simulink model "sampleModel68"  (R2021b)
settings: Solver=VariableStepAuto  StartTime=0.0  StopTime=10.0  RelTol=1e-3
undefined symbols (not defined in the file or in its folder): magnitude, Newton, Raphson
libraries: simulink x9, slpidlib x2
settings Model: Creator=user  LastModifiedBy=user

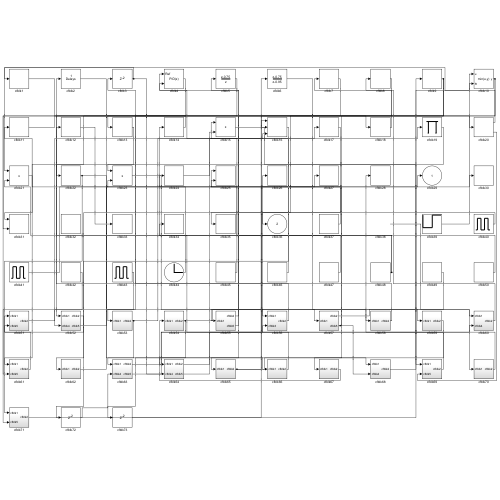
[thumbnail: Simulink's stored preview of the top-level diagram]
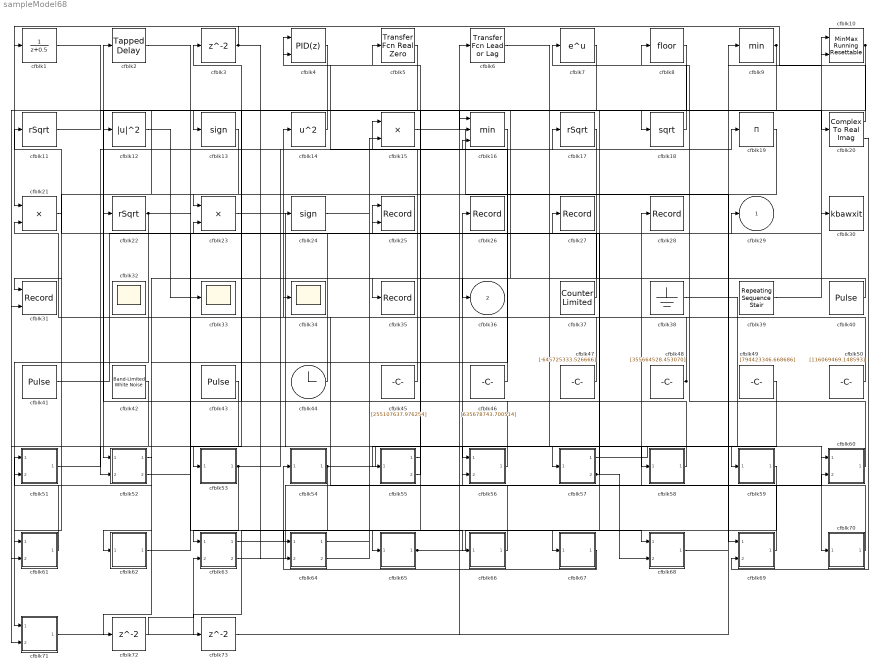
== system sampleModel68 ==
  cfblk1 : DiscreteTransferFcn  SampleTime=1
  cfblk10 : simulink/Math Operations/MinMax Running Resettable  Function=min  vinit=0.0
  cfblk11 : Sqrt  Operator=rSqrt  AlgorithmType=Newton-Raphson  SaturateOnIntegerOverflow=on
  cfblk12 : Math  Operator=magnitude^2  SaturateOnIntegerOverflow=on
  cfblk13 : Signum
  cfblk14 : Math  Operator=square  SaturateOnIntegerOverflow=on
  cfblk15 : Product  Inputs=**
  cfblk16 : MinMax  Inputs=3
  cfblk17 : Sqrt  Operator=rSqrt  AlgorithmType=Newton-Raphson  SaturateOnIntegerOverflow=on
  cfblk18 : Sqrt  SaturateOnIntegerOverflow=on
  cfblk19 : Product  Inputs=*
  cfblk2 : simulink/Discrete/Tapped Delay  vinit=0.0  samptime=-1  NumDelays=1  DelayOrder=Oldest  includeCurrent=off
  cfblk20 : ComplexToRealImag
  cfblk21 : Product
  cfblk22 : Sqrt  Operator=rSqrt  AlgorithmType=Newton-Raphson  SaturateOnIntegerOverflow=on
  cfblk23 : Product  Inputs=**
  cfblk24 : Signum
  cfblk25 : Record  FileSettingsInternal="{\"entries\":[{\"content\":{\"excelSettings\":{\"content\":{},\"type\":\"Streamout.ExcelSettings\"}},\"type\":\"Streamout.FileSettingStorage\",\"uuid\":\"7380ae25-d94a-4681-bf5d-5ee3cf68c672\"}],\"packageUris\":[\"http://schema.mathworks.com/mf0/streamout_blocks/R2020a\"],\"version\":\"1.0\"}"  Layout=[1 1]  SignalsInternal="{\"entries\":[{\"content\":{\"signals\":[{\"content\":{\"blockPath\":[\"sampleModel68/cfblk25\"],\"channel\":[],\"dimensions\":[1],\"domain\":\"sampleModel68/cfblk25\",\"lineColor\":\"#a2142f\",\"plots\":[1],\"port\":1,\"sid\":[\"\"],\"signalID\":2597,\"signalName\":\"cfblk45\"},\"type\":\"RecordBlkView.Signal\",\"uuid\":\"14372fe8-37bd-4dd9-b022-ca2b2938b13a\"},{\"content\":{\"blockPath\":[\"sampleModel68/cfblk25\"],\"channel\":[],\"dimensions\":[1],\"domain\":\"sampleModel68/cfblk25\",\"lineColor\":\"#139fff\",\"plots\":[1],\"port\":2,\"sid\":[\"\"],\"signalID\":2601,\"signalName\":\"cfblk57:2\"},\"type\":\"RecordBlkView.Signal\",\"uuid\":\"d926118c-bf66-4285-a082-df532e1a02d1\"}]},\"type\":\"RecordBlkView.InputSignals\",\"uuid\":\"7acbd860-2b2a-4c58-bd97-e2d0956e5af0\"}],\"packageUris\":[\"http://schema.mathworks.com/mf0/streamout_blocks/R2020a\"],\"version\":\"1.0\"}"  VisualizationBindings="{\"xyplotplugin\":{\"info\":[{\"series\":[{\"bindingParametersList\":[{\"parameter\":\"X-Axis\",\"signalID\":2597,\"signalName\":\"cfblk45\"},{\"parameter\":\"Y-Axis\",\"signalID\":2601,\"signalName\":\"cfblk57:2\"}],\"seriesID\":43011}],\"subplotID\":1}]}}"  CompatibilityTag=XY
  cfblk26 : Record  FileSettingsInternal="{\"entries\":[{\"content\":{\"excelSettings\":{\"content\":{},\"type\":\"Streamout.ExcelSettings\"}},\"type\":\"Streamout.FileSettingStorage\",\"uuid\":\"f47baa91-5e85-4539-9bdd-62570cf60bad\"}],\"packageUris\":[\"http://schema.mathworks.com/mf0/streamout_blocks/R2020a\"],\"version\":\"1.0\"}"  SignalsInternal="{\"entries\":[{\"content\":{\"signals\":[{\"content\":{\"blockPath\":[\"sampleModel68/cfblk26\"],\"channel\":[],\"dimensions\":[1],\"domain\":\"sampleModel68/cfblk26\",\"lineColor\":\"#0072bd\",\"plots\":[1],\"port\":1,\"sid\":[\"\"],\"signalID\":2617,\"signalName\":\"cfblk66\"},\"type\":\"RecordBlkView.Signal\",\"uuid\":\"ce7d10c1-a342-4b76-a021-8b8f96db9006\"}]},\"type\":\"RecordBlkView.InputSignals\",\"uuid\":\"a1fcf589-8043-40eb-83d7-4e4254cbec00\"}],\"packageUris\":[\"http://schema.mathworks.com/mf0/streamout_blocks/R2020a\"],\"version\":\"1.0\"}"  VisualizationBindings="{\"sparklinesplugin\":{\"info\":[{\"bindingParametersList\":[],\"subplotID\":1}]}}"
  cfblk27 : Record  FileSettingsInternal="{\"entries\":[{\"content\":{\"excelSettings\":{\"content\":{},\"type\":\"Streamout.ExcelSettings\"}},\"type\":\"Streamout.FileSettingStorage\",\"uuid\":\"7fca77e6-a95a-4af2-994f-8cefc4879576\"}],\"packageUris\":[\"http://schema.mathworks.com/mf0/streamout_blocks/R2020a\"],\"version\":\"1.0\"}"  SignalsInternal="{\"entries\":[{\"content\":{\"signals\":[{\"content\":{\"blockPath\":[\"sampleModel68/cfblk27\"],\"channel\":[],\"dimensions\":[1],\"domain\":\"sampleModel68/cfblk27\",\"lineColor\":\"#ff13a6\",\"plots\":[1],\"port\":1,\"sid\":[\"\"],\"signalID\":2605,\"signalName\":\"cfblk62\"},\"type\":\"RecordBlkView.Signal\",\"uuid\":\"25dd8e9c-f56c-4ed2-a9cf-a14533026692\"}]},\"type\":\"RecordBlkView.InputSignals\",\"uuid\":\"8aec1518-f338-4448-a462-eff875f2086d\"}],\"packageUris\":[\"http://schema.mathworks.com/mf0/streamout_blocks/R2020a\"],\"version\":\"1.0\"}"  VisualizationBindings="{\"sparklinesplugin\":{\"info\":[{\"bindingParametersList\":[],\"subplotID\":1}]}}"
  cfblk28 : Record  FileSettingsInternal="{\"entries\":[{\"content\":{\"excelSettings\":{\"content\":{},\"type\":\"Streamout.ExcelSettings\"}},\"type\":\"Streamout.FileSettingStorage\",\"uuid\":\"0b6a57c5-e48f-4051-9630-9944b72aff24\"}],\"packageUris\":[\"http://schema.mathworks.com/mf0/streamout_blocks/R2020a\"],\"version\":\"1.0\"}"  SignalsInternal="{\"entries\":[{\"content\":{\"signals\":[{\"content\":{\"blockPath\":[\"sampleModel68/cfblk28\"],\"channel\":[],\"dimensions\":[1],\"domain\":\"sampleModel68/cfblk28\",\"lineColor\":\"#edb120\",\"plots\":[1],\"port\":1,\"sid\":[\"\"],\"signalID\":2625,\"signalName\":\"cfblk70\"},\"type\":\"RecordBlkView.Signal\",\"uuid\":\"dc8e6425-624f-40ca-b929-8e8e8d4940ce\"}]},\"type\":\"RecordBlkView.InputSignals\",\"uuid\":\"d190679b-f694-456f-800b-168cbe042715\"}],\"packageUris\":[\"http://schema.mathworks.com/mf0/streamout_blocks/R2020a\"],\"version\":\"1.0\"}"  VisualizationBindings="{\"sparklinesplugin\":{\"info\":[{\"bindingParametersList\":[],\"subplotID\":1}]}}"
  cfblk3 : Delay  SampleTime=1
  cfblk30 : ToWorkspace  VariableName=kbawxit  SaveFormat=Timeseries  SampleTime=-1
  cfblk31 : Record  FileSettingsInternal="{\"entries\":[{\"content\":{\"excelSettings\":{\"content\":{},\"type\":\"Streamout.ExcelSettings\"}},\"type\":\"Streamout.FileSettingStorage\",\"uuid\":\"7dd7fc0f-01a8-4e3d-a00e-f98f5cc25ed7\"}],\"packageUris\":[\"http://schema.mathworks.com/mf0/streamout_blocks/R2020a\"],\"version\":\"1.0\"}"  Layout=[1 1]  SignalsInternal="{\"entries\":[{\"content\":{\"signals\":[{\"content\":{\"blockPath\":[\"sampleModel68/cfblk31\"],\"channel\":[],\"dimensions\":[1],\"domain\":\"sampleModel68/cfblk31\",\"lineColor\":\"#a2142f\",\"plots\":[1],\"port\":1,\"sid\":[\"\"],\"signalID\":2609,\"signalName\":\"cfblk13\"},\"type\":\"RecordBlkView.Signal\",\"uuid\":\"1befd8ad-63b6-41b6-b49e-12842e72401a\"},{\"content\":{\"blockPath\":[\"sampleModel68/cfblk31\"],\"channel\":[],\"dimensions\":[1],\"domain\":\"sampleModel68/cfblk31\",\"lineColor\":\"#139fff\",\"plots\":[1],\"port\":2,\"sid\":[\"\"],\"signalID\":2613,\"signalName\":\"cfblk4\"},\"type\":\"RecordBlkView.Signal\",\"uuid\":\"e4cc32b6-11bf-4c93-9d61-67df3e9ed535\"}]},\"type\":\"RecordBlkView.InputSignals\",\"uuid\":\"9e53f5fc-b0f2-4e3d-bb43-917b54e9e2d2\"}],\"packageUris\":[\"http://schema.mathworks.com/mf0/streamout_blocks/R2020a\"],\"version\":\"1.0\"}"  VisualizationBindings="{\"xyplotplugin\":{\"info\":[{\"series\":[{\"bindingParametersList\":[{\"parameter\":\"X-Axis\",\"signalID\":2609,\"signalName\":\"cfblk13\"},{\"parameter\":\"Y-Axis\",\"signalID\":2613,\"signalName\":\"cfblk4\"}],\"seriesID\":44428}],\"subplotID\":1}]}}"  CompatibilityTag=XY
  cfblk32 : Scope
      settings: Floating=on
  cfblk33 : Scope
  cfblk34 : Scope
  cfblk35 : Record  FileSettingsInternal="{\"entries\":[{\"content\":{\"excelSettings\":{\"content\":{},\"type\":\"Streamout.ExcelSettings\"}},\"type\":\"Streamout.FileSettingStorage\",\"uuid\":\"e62acdcb-7c93-4ae9-a251-67a68609c7cf\"}],\"packageUris\":[\"http://schema.mathworks.com/mf0/streamout_blocks/R2020a\"],\"version\":\"1.0\"}"  SignalsInternal="{\"entries\":[{\"content\":{\"signals\":[{\"content\":{\"blockPath\":[\"sampleModel68/cfblk35\"],\"channel\":[],\"dimensions\":[1],\"domain\":\"sampleModel68/cfblk35\",\"lineColor\":\"#d95319\",\"plots\":[1],\"port\":1,\"sid\":[\"\"],\"signalID\":2621,\"signalName\":\"cfblk40\"},\"type\":\"RecordBlkView.Signal\",\"uuid\":\"cba5933c-5ebb-4ff9-ad8b-2eadd83d23f5\"}]},\"type\":\"RecordBlkView.InputSignals\",\"uuid\":\"4eef4586-6a89-45b6-bd2f-dfe3524fb43a\"}],\"packageUris\":[\"http://schema.mathworks.com/mf0/streamout_blocks/R2020a\"],\"version\":\"1.0\"}"  VisualizationBindings="{\"sparklinesplugin\":{\"info\":[{\"bindingParametersList\":[],\"subplotID\":1}]}}"
  cfblk37 : simulink/Sources/Counter Limited  uplimit=[649.000000]  tsamp=-1
  cfblk38 : Ground
  cfblk39 : simulink/Sources/Repeating Sequence Stair  OutValues=[645973491.139830, 703038970.892550]  tsamp=-1  OutMin=[]  OutMax=[]  OutDataTypeStr=double  OutputDataTypeScalingMode=double  OutDataType=fixdt(0,8)  ConRadixGroup=Best Precision: Vector-wise  OutScaling=2^-12
  cfblk4 : slpidlib/PID Controller (2DOF)  Controller=PID  Form=Parallel  TimeDomain=Discrete-time  UseExternalTs=off  SampleTime=1  IntegratorMethod=Forward Euler  FilterMethod=Forward Euler  ControllerParametersSource=internal  P=1  I=1  D=0  UseFilter=on  N=100  b=1  c=1  TunerSelectOption=Transfer Function Based (PID Tuner App)  InitialConditionSource=internal  InitialConditionForIntegrator=0  InitialConditionForFilter=0  DifferentiatorICPrevScaledInput=0  ExternalReset=none  TrackingMode=off  Kt=1  LimitOutput=off  SatLimitsSource=internal  UpperSaturationLimit=inf  LowerSaturationLimit=-inf  LinearizeAsGain=off  AntiWindupMode=none  Kb=1  POutMin=[]  POutMax=[]  IOutMin=[]  IOutMax=[]  DOutMin=[]  DOutMax=[]  NOutMin=[]  NOutMax=[]  bOutMin=[]  bOutMax=[]  cOutMin=[]  cOutMax=[]  SumOutMin=[]  SumOutMax=[]  SaturationOutMin=[]  SaturationOutMax=[]  PParamMin=[]  PParamMax=[]  IParamMin=[]  IParamMax=[]  DParamMin=[]  DParamMax=[]  NParamMin=[]  NParamMax=[]  bParamMin=[]  bParamMax=[]  cParamMin=[]  cParamMax=[]  KbParamMin=[]  KbParamMax=[]  KtParamMin=[]  KtParamMax=[]  KbOutMin=[]  KbOutMax=[]  KtOutMin=[]  KtOutMax=[]  IntegratorOutMin=[]  IntegratorOutMax=[]  FilterOutMin=[]  FilterOutMax=[]  SumI1OutMin=[]  SumI1OutMax=[]  SumI2OutMin=[]  SumI2OutMax=[]  SumI3OutMin=[]  SumI3OutMax=[]  SumI4OutMin=[]  SumI4OutMax=[]  SumDOutMin=[]  SumDOutMax=[]  Sum1OutMin=[]  Sum1OutMax=[]  Sum2OutMin=[]  Sum2OutMax=[]  Sum3OutMin=[]  Sum3OutMax=[]  DifferentiatorOutMin=[]  DifferentiatorOutMax=[]  FilterDiffOutCoefMin=[]  FilterDiffOutCoefMax=[]  ReciprocalOutMin=[]  ReciprocalOutMax=[]  SumDenOutMin=[]  SumDenOutMax=[]  SumNumOutMin=[]  SumNumOutMax=[]  DivideOutMin=[]  DivideOutMax=[]  UdiffTsProdOutMin=[]  UdiffTsProdOutMax=[]  NTsProdOutMin=[]  NTsProdOutMax=[]  UintegralTsProdOutMin=[]  UintegralTsProdOutMax=[]  UngainTsProdOutMin=[]  UngainTsProdOutMax=[]  IntegratorContinuousStateAttributes=''  IntegratorStateMustResolveToSignalObject=off  IntegratorRTWStateStorageClass=Auto  FilterContinuousStateAttributes=''  FilterStateMustResolveToSignalObject=off  FilterRTWStateStorageClass=Auto  ParallelPVariant=InternalParameters  IdealPVariant=Disabled  IVariant=InternalParameters  DVariant=InternalParameters  bVariant=InternalParameters  cVariant=InternalParameters  IntegratorVariant=Discrete  SatVariant=Disabled  AWVariant=Passthrough  PCopyVariant=Disabled  TRVariant=Disabled  FdbkBlocksVariant=Forward  IdealPFdbkVariant=Disabled  SatFdbkVariant=Disabled  DerivativeFilterVariant=ForwardEulerFilter  NVariant=InternalParameters  NCopyVariant=Disabled  FilterICVariant=InternalICsFilter  IntegratorICVariant=InternalICs  ExternalResetVariant=Disabled  TRSumVariant=Passthrough  SumFdbkVariant=Disabled  SumVariant=Sum_PID  TsampFilterVariant=InternalTs  TsampNgainVariant=Passthrough  TsampIntegralVariant=Passthrough  ExternalSaturationOutDataTypeStr=Inherit: Same as second input
      settings: SourceProductBaseCode=SL
  cfblk40 : DiscretePulseGenerator  PulseType=Time based  Amplitude=[-445442640.127411]  Period=[11449827.973829]  PulseWidth=5  PhaseDelay=[6.000000]
  cfblk41 : DiscretePulseGenerator  PulseType=Time based  Amplitude=[-687630750.798750]  Period=[5327849.825297]  PulseWidth=5  PhaseDelay=[4.000000]
  cfblk42 : simulink/Sources/Band-Limited White Noise  Cov=[9357779221.486231]  Ts=0.1  seed=[2033079699.000000]
  cfblk43 : DiscretePulseGenerator  PulseType=Time based  Amplitude=[-140736143.976516]  Period=[50342523.627179]  PulseWidth=5  PhaseDelay=[2.000000]
  cfblk44 : Clock
  cfblk45 : Constant  Value=[255107637.976254]  SampleTime=1
  cfblk46 : Constant  Value=[635678743.700514]  SampleTime=1
  cfblk47 : Constant  Value=[-645725333.526666]  SampleTime=1
  cfblk48 : Constant  Value=[355664528.453070]  SampleTime=1
  cfblk49 : Constant  Value=[794423346.668686]  SampleTime=1
  cfblk5 : simulink/Discrete/Transfer Fcn Real Zero  ZeroZ=0.75  ICPrevInput=0.0  DoSatur=off
      settings: SourceProductBaseCode=SL
  cfblk50 : Constant  Value=[116069469.148593]  SampleTime=1
  cfblk51 : Subsystem
  cfblk52 : Subsystem
  cfblk53 : Subsystem
  cfblk54 : Subsystem
  cfblk55 : Subsystem
  cfblk56 : Subsystem
  cfblk57 : Subsystem
  cfblk58 : Subsystem
  cfblk59 : Subsystem
  cfblk6 : simulink/Discrete/Transfer Fcn Lead or Lag  PoleZ=0.95  ZeroZ=0.75  ICPrevOutput=0.0  ICPrevInput=0.0  DoSatur=off
      settings: SourceProductBaseCode=SL
  cfblk60 : Subsystem
  cfblk61 : Subsystem
  cfblk62 : Subsystem
  cfblk63 : Subsystem
  cfblk64 : Subsystem
  cfblk65 : Subsystem
  cfblk66 : Subsystem
  cfblk67 : Subsystem
  cfblk68 : Subsystem
  cfblk69 : Subsystem
  cfblk7 : Math  SaturateOnIntegerOverflow=on
  cfblk70 : Subsystem
  cfblk71 : Subsystem
  cfblk72 : Delay  SampleTime=1
  cfblk73 : Delay  SampleTime=1
  cfblk8 : Rounding
  cfblk9 : MinMax
  cfblk29 : Outport
  cfblk36 : Outport  Port=2
  wires:
  cfblk40/1 -> cfblk35/1
  cfblk66/1(cfblk2) -> cfblk26/1
  cfblk67/1(cfblk2) -> cfblk54/1(cfblk1)
  cfblk12/1 -> cfblk33/1
  cfblk48/1 -> cfblk15/1, cfblk21/2
  cfblk20/1 -> cfblk21/1
  cfblk56/1(cfblk2) -> cfblk2/1
  cfblk50/1 -> cfblk14/1
  cfblk54/1(cfblk2) -> cfblk59/1(cfblk1), cfblk64/1(cfblk1)
  cfblk53/1(cfblk2) -> cfblk63/1(cfblk1), cfblk16/3
  cfblk5/1 -> cfblk52/1(cfblk1)
  cfblk22/1 -> cfblk71/1(cfblk1), cfblk57/1(cfblk1)
  cfblk55/1(cfblk2) -> cfblk5/1
  cfblk42/1 -> cfblk71/2(cfblk5)
  cfblk9/1 -> cfblk36/1, cfblk22/1, cfblk61/2(cfblk5)
  cfblk43/1 -> cfblk52/2(cfblk4)
  cfblk51/1(cfblk2) -> cfblk17/1
  cfblk38/1 -> cfblk70/1(cfblk1)
  cfblk47/1 -> cfblk12/1
  cfblk23/1 -> cfblk56/1(cfblk1)
  cfblk71/1(cfblk2) -> cfblk6/1
  cfblk58/1(cfblk2) -> cfblk3/1
  cfblk69/1(cfblk2) -> cfblk34/1
  cfblk37/1 -> cfblk24/1
  cfblk17/1 -> cfblk62/1(cfblk1)
  cfblk44/1 -> cfblk11/1
  cfblk61/1(cfblk2) -> cfblk51/1(cfblk1)
  cfblk15/1 -> cfblk69/1(cfblk1)
  cfblk3/1 -> cfblk1/1, cfblk64/2(cfblk4)
  cfblk70/1(cfblk2) -> cfblk28/1
  cfblk18/1 -> cfblk7/1
  cfblk63/1(cfblk2) -> cfblk16/1
  cfblk63/2(cfblk5) -> cfblk56/2(cfblk3)
  cfblk21/1 -> cfblk61/1(cfblk1)
  cfblk39/1 -> cfblk10/1
  cfblk45/1 -> cfblk25/1
  cfblk65/1(cfblk2) -> cfblk68/1(cfblk1), cfblk29/1
  cfblk20/2 -> cfblk69/2(cfblk5)
  cfblk6/1 -> cfblk58/1(cfblk1)
  cfblk8/1 -> cfblk16/2
  cfblk2/1 -> cfblk66/1(cfblk1)
  cfblk10/1 -> cfblk55/1(cfblk1), cfblk67/1(cfblk1)
  cfblk57/1(cfblk2) -> cfblk60/1(cfblk1)
  cfblk11/1 -> cfblk20/1
  cfblk64/1(cfblk2) -> cfblk15/2
  cfblk7/1 -> cfblk53/1(cfblk1)
  cfblk13/1 -> cfblk31/1
  cfblk60/1(cfblk2) -> cfblk8/1
  cfblk1/1 -> cfblk18/1
  cfblk46/1 -> cfblk4/1
  cfblk4/1 -> cfblk31/2
  cfblk55/2(cfblk5) -> cfblk4/2
  cfblk19/1 -> cfblk23/1
  cfblk52/1(cfblk2) -> cfblk51/2(cfblk5)
  cfblk49/1 -> cfblk65/1(cfblk1)
  cfblk68/1(cfblk2) -> cfblk10/2
  cfblk14/1 -> cfblk13/1
  cfblk62/1(cfblk2) -> cfblk27/1
  cfblk57/2(cfblk5) -> cfblk25/2, cfblk68/2(cfblk4)
  cfblk41/1 -> cfblk23/2
  cfblk64/2(cfblk5) -> cfblk60/2(cfblk4)
  cfblk24/1 -> cfblk19/1
  cfblk52/2(cfblk5) -> cfblk30/1
  cfblk16/1 -> cfblk72/1
  cfblk72/1 -> cfblk63/2(cfblk4)
  cfblk59/1(cfblk2) -> cfblk73/1
  cfblk73/1 -> cfblk9/1

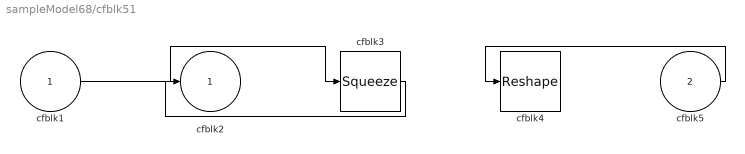
== system sampleModel68/cfblk51 ==
  cfblk1 : Inport
  cfblk5 : Inport  Port=2
  cfblk3 : Squeeze
  cfblk4 : Reshape
  cfblk2 : Outport
  wires:
  cfblk1/1 -> cfblk3/1
  cfblk5/1 -> cfblk4/1
  cfblk3/1 -> cfblk2/1

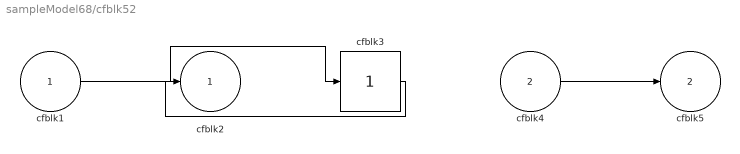
== system sampleModel68/cfblk52 ==
  cfblk1 : Inport
  cfblk4 : Inport  Port=2
  cfblk3 : simulink/Math Operations/Slider Gain  gain=1  low=0  high=2
  cfblk2 : Outport
  cfblk5 : Outport  Port=2
  wires:
  cfblk4/1 -> cfblk5/1
  cfblk1/1 -> cfblk3/1
  cfblk3/1 -> cfblk2/1

== system sampleModel68/cfblk53 ==
  cfblk1 : Inport
  cfblk3 : Delay  SampleTime=1
  cfblk2 : Outport
  wires:
  cfblk1/1 -> cfblk3/1
  cfblk3/1 -> cfblk2/1

== system sampleModel68/cfblk54 ==
  cfblk1 : Inport
  cfblk3 : DiscreteTransferFcn  SampleTime=1
  cfblk2 : Outport
  wires:
  cfblk3/1 -> cfblk2/1
  cfblk1/1 -> cfblk3/1

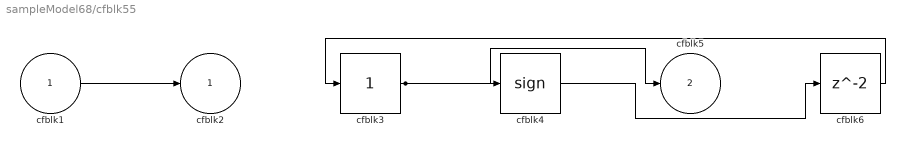
== system sampleModel68/cfblk55 ==
  cfblk1 : Inport
  cfblk3 : simulink/Math Operations/Slider Gain  gain=1  low=0  high=2
  cfblk4 : Signum
  cfblk6 : Delay  SampleTime=1
  cfblk2 : Outport
  cfblk5 : Outport  Port=2
  wires:
  cfblk1/1 -> cfblk2/1
  cfblk3/1 -> cfblk5/1, cfblk4/1
  cfblk4/1 -> cfblk6/1
  cfblk6/1 -> cfblk3/1

== system sampleModel68/cfblk56 ==
  cfblk1 : Inport
  cfblk3 : Inport  Port=2
  cfblk2 : Outport
  wires:
  cfblk1/1 -> cfblk2/1

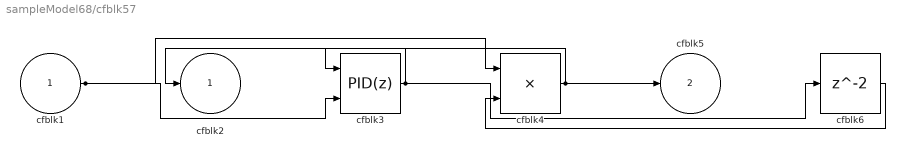
== system sampleModel68/cfblk57 ==
  cfblk1 : Inport
  cfblk3 : slpidlib/PID Controller (2DOF)  Controller=PID  Form=Parallel  TimeDomain=Discrete-time  UseExternalTs=off  SampleTime=1  IntegratorMethod=Forward Euler  FilterMethod=Forward Euler  ControllerParametersSource=internal  P=1  I=1  D=0  UseFilter=on  N=100  b=1  c=1  TunerSelectOption=Transfer Function Based (PID Tuner App)  InitialConditionSource=internal  InitialConditionForIntegrator=0  InitialConditionForFilter=0  DifferentiatorICPrevScaledInput=0  ExternalReset=none  TrackingMode=off  Kt=1  LimitOutput=off  SatLimitsSource=internal  UpperSaturationLimit=inf  LowerSaturationLimit=-inf  LinearizeAsGain=off  AntiWindupMode=none  Kb=1  POutMin=[]  POutMax=[]  IOutMin=[]  IOutMax=[]  DOutMin=[]  DOutMax=[]  NOutMin=[]  NOutMax=[]  bOutMin=[]  bOutMax=[]  cOutMin=[]  cOutMax=[]  SumOutMin=[]  SumOutMax=[]  SaturationOutMin=[]  SaturationOutMax=[]  PParamMin=[]  PParamMax=[]  IParamMin=[]  IParamMax=[]  DParamMin=[]  DParamMax=[]  NParamMin=[]  NParamMax=[]  bParamMin=[]  bParamMax=[]  cParamMin=[]  cParamMax=[]  KbParamMin=[]  KbParamMax=[]  KtParamMin=[]  KtParamMax=[]  KbOutMin=[]  KbOutMax=[]  KtOutMin=[]  KtOutMax=[]  IntegratorOutMin=[]  IntegratorOutMax=[]  FilterOutMin=[]  FilterOutMax=[]  SumI1OutMin=[]  SumI1OutMax=[]  SumI2OutMin=[]  SumI2OutMax=[]  SumI3OutMin=[]  SumI3OutMax=[]  SumI4OutMin=[]  SumI4OutMax=[]  SumDOutMin=[]  SumDOutMax=[]  Sum1OutMin=[]  Sum1OutMax=[]  Sum2OutMin=[]  Sum2OutMax=[]  Sum3OutMin=[]  Sum3OutMax=[]  DifferentiatorOutMin=[]  DifferentiatorOutMax=[]  FilterDiffOutCoefMin=[]  FilterDiffOutCoefMax=[]  ReciprocalOutMin=[]  ReciprocalOutMax=[]  SumDenOutMin=[]  SumDenOutMax=[]  SumNumOutMin=[]  SumNumOutMax=[]  DivideOutMin=[]  DivideOutMax=[]  UdiffTsProdOutMin=[]  UdiffTsProdOutMax=[]  NTsProdOutMin=[]  NTsProdOutMax=[]  UintegralTsProdOutMin=[]  UintegralTsProdOutMax=[]  UngainTsProdOutMin=[]  UngainTsProdOutMax=[]  IntegratorContinuousStateAttributes=''  IntegratorStateMustResolveToSignalObject=off  IntegratorRTWStateStorageClass=Auto  FilterContinuousStateAttributes=''  FilterStateMustResolveToSignalObject=off  FilterRTWStateStorageClass=Auto  ParallelPVariant=InternalParameters  IdealPVariant=Disabled  IVariant=InternalParameters  DVariant=InternalParameters  bVariant=InternalParameters  cVariant=InternalParameters  IntegratorVariant=Discrete  SatVariant=Disabled  AWVariant=Passthrough  PCopyVariant=Disabled  TRVariant=Disabled  FdbkBlocksVariant=Forward  IdealPFdbkVariant=Disabled  SatFdbkVariant=Disabled  DerivativeFilterVariant=ForwardEulerFilter  NVariant=InternalParameters  NCopyVariant=Disabled  FilterICVariant=InternalICsFilter  IntegratorICVariant=InternalICs  ExternalResetVariant=Disabled  TRSumVariant=Passthrough  SumFdbkVariant=Disabled  SumVariant=Sum_PID  TsampFilterVariant=InternalTs  TsampNgainVariant=Passthrough  TsampIntegralVariant=Passthrough  ExternalSaturationOutDataTypeStr=Inherit: Same as second input
      settings: SourceProductBaseCode=SL
  cfblk4 : Product
  cfblk6 : Delay  SampleTime=1
  cfblk2 : Outport
  cfblk5 : Outport  Port=2
  wires:
  cfblk3/1 -> cfblk2/1, cfblk6/1
  cfblk1/1 -> cfblk4/1, cfblk3/2
  cfblk4/1 -> cfblk5/1, cfblk3/1
  cfblk6/1 -> cfblk4/2

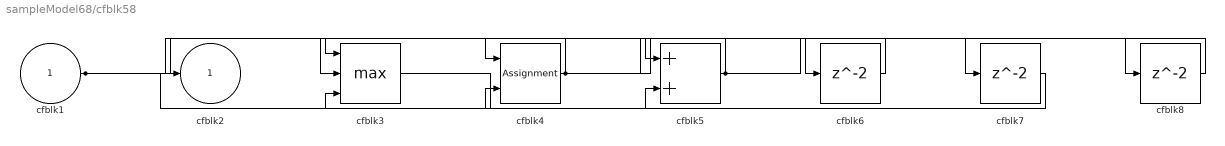
== system sampleModel68/cfblk58 ==
  cfblk1 : Inport
  cfblk3 : MinMax  Function=max  Inputs=3
  cfblk4 : Assignment  DiagnosticForDimensions=Warning  IndexOptions=Index vector (dialog)  Indices=1  OutputSizes=1
  cfblk5 : Sum
  cfblk6 : Delay  SampleTime=1
  cfblk7 : Delay  SampleTime=1
  cfblk8 : Delay  SampleTime=1
  cfblk2 : Outport
  wires:
  cfblk4/1 -> cfblk2/1, cfblk6/1, cfblk7/1
  cfblk1/1 -> cfblk3/1, cfblk4/2
  cfblk3/1 -> cfblk5/2
  cfblk5/1 -> cfblk4/1, cfblk8/1
  cfblk6/1 -> cfblk5/1
  cfblk7/1 -> cfblk3/3
  cfblk8/1 -> cfblk3/2

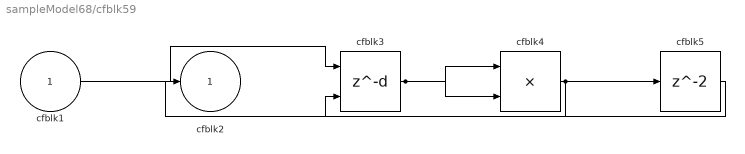
== system sampleModel68/cfblk59 ==
  cfblk1 : Inport
  cfblk3 : Delay  DelayLengthSource=Input port  SampleTime=1
      settings: InputPortMap=u0,p1
  cfblk4 : Product
  cfblk5 : Delay  SampleTime=1
  cfblk2 : Outport
  wires:
  cfblk1/1 -> cfblk3/1
  cfblk3/1 -> cfblk4/1, cfblk4/2
  cfblk4/1 -> cfblk2/1, cfblk5/1
  cfblk5/1 -> cfblk3/2

== system sampleModel68/cfblk60 ==
  cfblk1 : Inport
  cfblk4 : Inport  Port=2
  cfblk3 : Constant  Value=[829645821.804819]  SampleTime=1
  cfblk2 : Outport
  wires:
  cfblk4/1 -> cfblk2/1

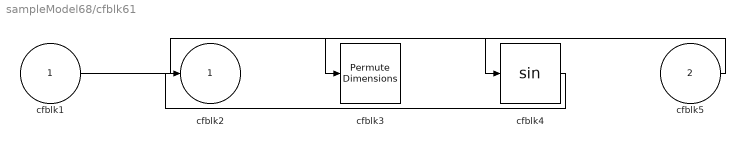
== system sampleModel68/cfblk61 ==
  cfblk1 : Inport
  cfblk5 : Inport  Port=2
  cfblk3 : PermuteDimensions
  cfblk4 : Trigonometry
  cfblk2 : Outport
  wires:
  cfblk1/1 -> cfblk4/1
  cfblk4/1 -> cfblk2/1
  cfblk5/1 -> cfblk3/1

== system sampleModel68/cfblk62 ==
  cfblk1 : Inport
  cfblk3 : UnaryMinus
  cfblk2 : Outport
  wires:
  cfblk1/1 -> cfblk2/1, cfblk3/1

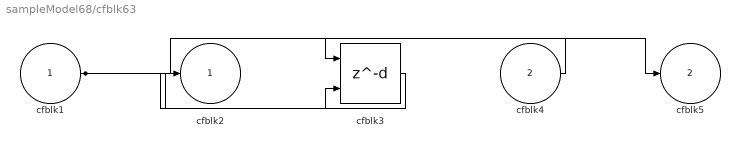
== system sampleModel68/cfblk63 ==
  cfblk1 : Inport
  cfblk4 : Inport  Port=2
  cfblk3 : Delay  DelayLengthSource=Input port  SampleTime=1
      settings: InputPortMap=u0,p1
  cfblk2 : Outport
  cfblk5 : Outport  Port=2
  wires:
  cfblk1/1 -> cfblk5/1, cfblk3/2
  cfblk3/1 -> cfblk2/1
  cfblk4/1 -> cfblk3/1

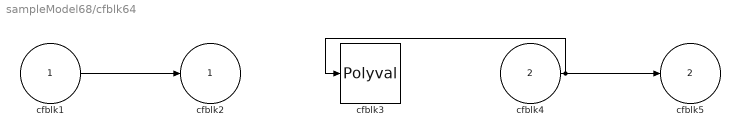
== system sampleModel68/cfblk64 ==
  cfblk1 : Inport
  cfblk4 : Inport  Port=2
  cfblk3 : Polyval  Coefs=[ +2.081618890e-019, -1.441693666e-014, +4.719686976e-010, -8.536869453e-006, +1.621573104e-001, -8.087801117e+001 ]
  cfblk2 : Outport
  cfblk5 : Outport  Port=2
  wires:
  cfblk1/1 -> cfblk2/1
  cfblk4/1 -> cfblk5/1, cfblk3/1

== system sampleModel68/cfblk65 ==
  cfblk1 : Inport
  cfblk3 : Assignment  DiagnosticForDimensions=Warning  IndexOptions=Index vector (dialog)  Indices=1  OutputSizes=1
  cfblk2 : Outport
  wires:
  cfblk3/1 -> cfblk2/1
  cfblk1/1 -> cfblk3/1, cfblk3/2

== system sampleModel68/cfblk66 ==
  cfblk1 : Inport
  cfblk3 : Gain  Gain=[-285234666.577093]
  cfblk2 : Outport
  wires:
  cfblk1/1 -> cfblk3/1
  cfblk3/1 -> cfblk2/1

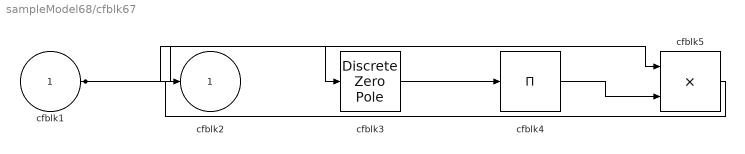
== system sampleModel68/cfblk67 ==
  cfblk1 : Inport
  cfblk3 : DiscreteZeroPole  Poles=[0 0.5]  Gain=1
  cfblk4 : Product  Inputs=*
  cfblk5 : Product  Inputs=**
  cfblk2 : Outport
  wires:
  cfblk1/1 -> cfblk5/1, cfblk3/1
  cfblk5/1 -> cfblk2/1
  cfblk3/1 -> cfblk4/1
  cfblk4/1 -> cfblk5/2

== system sampleModel68/cfblk68 ==
  cfblk1 : Inport
  cfblk4 : Inport  Port=2
  cfblk3 : Squeeze
  cfblk2 : Outport
  wires:
  cfblk4/1 -> cfblk3/1
  cfblk3/1 -> cfblk2/1

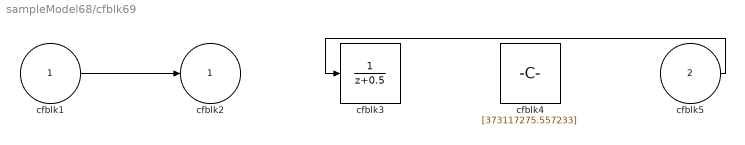
== system sampleModel68/cfblk69 ==
  cfblk1 : Inport
  cfblk5 : Inport  Port=2
  cfblk3 : DiscreteTransferFcn  SampleTime=1
  cfblk4 : Constant  Value=[373117275.557233]  SampleTime=1
  cfblk2 : Outport
  wires:
  cfblk1/1 -> cfblk2/1
  cfblk5/1 -> cfblk3/1

== system sampleModel68/cfblk70 ==
  cfblk1 : Inport
  cfblk3 : Math  Operator=square  SaturateOnIntegerOverflow=on
  cfblk2 : Outport
  wires:
  cfblk1/1 -> cfblk2/1, cfblk3/1

== system sampleModel68/cfblk71 ==
  cfblk1 : Inport
  cfblk5 : Inport  Port=2
  cfblk3 : DiscreteTransferFcn  SampleTime=1
  cfblk4 : Sum  Inputs=|++
  cfblk2 : Outport
  wires:
  cfblk5/1 -> cfblk3/1
  cfblk1/1 -> cfblk4/1
  cfblk4/1 -> cfblk2/1
  cfblk3/1 -> cfblk4/2
